simulink model "blockset_Q36121333"  (R2023a)
settings: Solver=VariableStepAuto  StartTime=0.0  StopTime=0.002  FixedStep=2e-12  MaxStep=1e-7  RelTol=1e-3
undefined symbols (not defined in the file or in its folder): plecs
libraries: plecslib_extras2 x5, simulink x5
settings Model: Creator=stanl  LastModifiedBy=stanl
settings SolverCC: ConsecutiveZCsStepRelTol=10*1280*eps
settings DataIOCC: ReturnWorkspaceOutputs=off

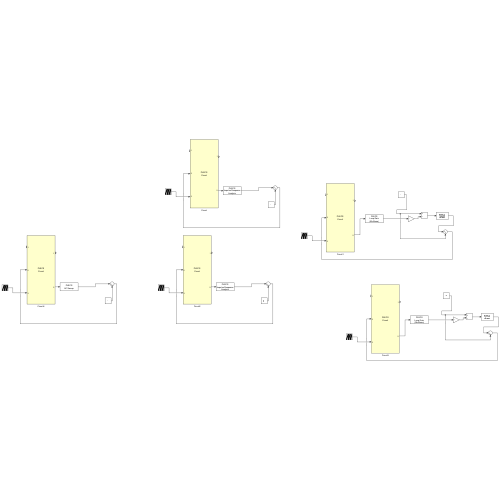
[thumbnail: Simulink's stored preview of the top-level diagram]
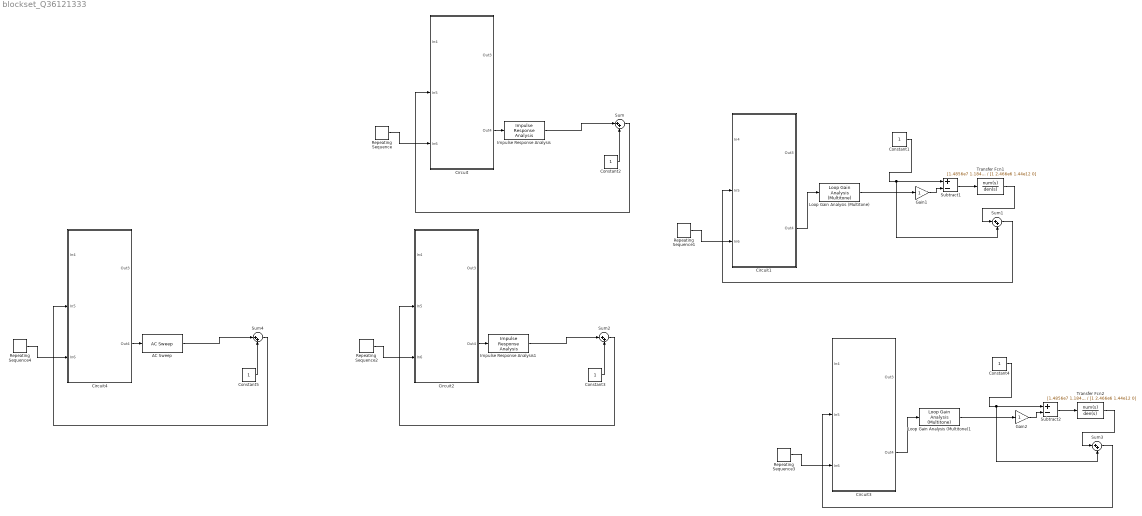
== system blockset_Q36121333 ==
  AC Sweep : plecslib_extras2/Analysis Tools/AC Sweep  FreqRange=[100 500000]  FreqScale=logarithmic  NPoints=21  InitialAmplitude=1e-3  TimeSpan=2e-6  TStart=0  ShowRefInput=off  Method=Steady-state analysis - start from model initial state  MaxIter=20  Tolerance=1e-4  Display=final  HideScopes=off  HiddenStates=error  OutputName=T  BodePlot=on  JPert=1e-4  NInitCycles=0
      settings: SourceProductName=PLECS Extras
  Circuit : Subsystem  LoadFcn=plecs('sl', 200);  InitFcn=plecs('sl', 214);  StartFcn=plecs('sl', 208);  StopFcn=plecs('sl', 209);  mask(PlecsCircuit){PLECSData=<binary blob, 3108 chars, not shown>}
      mask prompts: PLECSData "PLECS Data (Do not delete or modify!)"
      mask init:
      | % PLACE CUSTOM INITIALIZATIONS ABOVE
      | % DO NOT REMOVE
      | plecs('sl', 215);
      | % DO NOT REMOVE
      settings: CopyFcn=plecs('sl', 203);  DeleteFcn=plecs('sl', 205);  UndoDeleteFcn=plecs('sl', 206);  PreSaveFcn=plecs('sl', 211);  PostSaveFcn=plecs('sl', 201);  NameChangeFcn=plecs('sl', 210);  DestroyFcn=plecs('sl', 207);  PreCopyFcn=plecs('sl', 216);  OpenFcn=plecs('sl', 202);  ErrorFcn=plerrorfcn
      mask Help: web(['file:///' fullfile(plecsdoc, 'creatingacircuit.html')])
      mask Display: disp('PLECS\nCircuit')
  Circuit1 : Subsystem  LoadFcn=plecs('sl', 200);  InitFcn=plecs('sl', 214);  StartFcn=plecs('sl', 208);  StopFcn=plecs('sl', 209);  mask(PlecsCircuit){PLECSData=<binary blob, 3100 chars, not shown>}
      mask prompts: PLECSData "PLECS Data (Do not delete or modify!)"
      mask init:
      | % PLACE CUSTOM INITIALIZATIONS ABOVE
      | % DO NOT REMOVE
      | plecs('sl', 215);
      | % DO NOT REMOVE
      settings: CopyFcn=plecs('sl', 203);  DeleteFcn=plecs('sl', 205);  UndoDeleteFcn=plecs('sl', 206);  PreSaveFcn=plecs('sl', 211);  PostSaveFcn=plecs('sl', 201);  NameChangeFcn=plecs('sl', 210);  DestroyFcn=plecs('sl', 207);  PreCopyFcn=plecs('sl', 216);  OpenFcn=plecs('sl', 202);  ErrorFcn=plerrorfcn
      mask Help: web(['file:///' fullfile(plecsdoc, 'creatingacircuit.html')])
      mask Display: disp('PLECS\nCircuit')
  Circuit2 : Subsystem  LoadFcn=plecs('sl', 200);  InitFcn=plecs('sl', 214);  StartFcn=plecs('sl', 208);  StopFcn=plecs('sl', 209);  mask(PlecsCircuit){PLECSData=<binary blob, 3112 chars, not shown>}
      mask prompts: PLECSData "PLECS Data (Do not delete or modify!)"
      mask init:
      | % PLACE CUSTOM INITIALIZATIONS ABOVE
      | % DO NOT REMOVE
      | plecs('sl', 215);
      | % DO NOT REMOVE
      settings: CopyFcn=plecs('sl', 203);  DeleteFcn=plecs('sl', 205);  UndoDeleteFcn=plecs('sl', 206);  PreSaveFcn=plecs('sl', 211);  PostSaveFcn=plecs('sl', 201);  NameChangeFcn=plecs('sl', 210);  DestroyFcn=plecs('sl', 207);  PreCopyFcn=plecs('sl', 216);  OpenFcn=plecs('sl', 202);  ErrorFcn=plerrorfcn
      mask Help: web(['file:///' fullfile(plecsdoc, 'creatingacircuit.html')])
      mask Display: disp('PLECS\nCircuit')
  Circuit3 : Subsystem  LoadFcn=plecs('sl', 200);  InitFcn=plecs('sl', 214);  StartFcn=plecs('sl', 208);  StopFcn=plecs('sl', 209);  mask(PlecsCircuit){PLECSData=<binary blob, 3096 chars, not shown>}
      mask prompts: PLECSData "PLECS Data (Do not delete or modify!)"
      mask init:
      | % PLACE CUSTOM INITIALIZATIONS ABOVE
      | % DO NOT REMOVE
      | plecs('sl', 215);
      | % DO NOT REMOVE
      settings: CopyFcn=plecs('sl', 203);  DeleteFcn=plecs('sl', 205);  UndoDeleteFcn=plecs('sl', 206);  PreSaveFcn=plecs('sl', 211);  PostSaveFcn=plecs('sl', 201);  NameChangeFcn=plecs('sl', 210);  DestroyFcn=plecs('sl', 207);  PreCopyFcn=plecs('sl', 216);  OpenFcn=plecs('sl', 202);  ErrorFcn=plerrorfcn
      mask Help: web(['file:///' fullfile(plecsdoc, 'creatingacircuit.html')])
      mask Display: disp('PLECS\nCircuit')
  Circuit4 : Subsystem  LoadFcn=plecs('sl', 200);  InitFcn=plecs('sl', 214);  StartFcn=plecs('sl', 208);  StopFcn=plecs('sl', 209);  mask(PlecsCircuit){PLECSData=<binary blob, 3104 chars, not shown>}
      mask prompts: PLECSData "PLECS Data (Do not delete or modify!)"
      mask init:
      | % PLACE CUSTOM INITIALIZATIONS ABOVE
      | % DO NOT REMOVE
      | plecs('sl', 215);
      | % DO NOT REMOVE
      settings: CopyFcn=plecs('sl', 203);  DeleteFcn=plecs('sl', 205);  UndoDeleteFcn=plecs('sl', 206);  PreSaveFcn=plecs('sl', 211);  PostSaveFcn=plecs('sl', 201);  NameChangeFcn=plecs('sl', 210);  DestroyFcn=plecs('sl', 207);  PreCopyFcn=plecs('sl', 216);  OpenFcn=plecs('sl', 202);  ErrorFcn=plerrorfcn
      mask Help: web(['file:///' fullfile(plecsdoc, 'creatingacircuit.html')])
      mask Display: disp('PLECS\nCircuit')
  Constant{1..5} (5 alike) : Constant
  Gain1 : Gain
  Gain2 : Gain
  Impulse Response Analysis : plecslib_extras2/Analysis Tools/Impulse Response Analysis  FreqRange=[100 200000]  FreqScale=logarithmic  NPoints=300  Perturbation=1e-3  Compensation=discrete pulse  TimeSpan=2e-6  TStart=0  MaxIter=20  Tolerance=1e-6  Display=iteration  HideScopes=on  HiddenStates=error  OutputName=T  BodePlot=on  JPert=1e-4  NInitCycles=0
      settings: SourceProductName=PLECS Extras
  Impulse Response Analysis1 : plecslib_extras2/Analysis Tools/Impulse Response Analysis  FreqRange=[100 200000]  FreqScale=logarithmic  NPoints=300  Perturbation=1e-3  Compensation=discrete pulse  TimeSpan=2e-6  TStart=0  MaxIter=20  Tolerance=1e-6  Display=iteration  HideScopes=on  HiddenStates=error  OutputName=T  BodePlot=on  JPert=1e-4  NInitCycles=0
      settings: SourceProductName=PLECS Extras
  Loop Gain Analysis (Multitone) : plecslib_extras2/Analysis Tools/Loop Gain Analysis (Multitone)  FreqRange=[100 200000]  Amplitude=1e-3  TStart=0.02  Display=final  HideScopes=off  OutputName=T  BodePlot=on
      settings: SourceProductName=PLECS Extras
  Loop Gain Analysis (Multitone)1 : plecslib_extras2/Analysis Tools/Loop Gain Analysis (Multitone)  FreqRange=[100 200000]  Amplitude=1e-3  TStart=0.02  Display=final  HideScopes=off  OutputName=T  BodePlot=on
      settings: SourceProductName=PLECS Extras
  Repeating Sequence{,1..4} (5 alike) : simulink/Sources/Repeating Sequence  rep_seq_t=[0 2e-6]  rep_seq_y=[0 3]
  Subtract1 : Sum  Inputs=+-
  Subtract2 : Sum  Inputs=+-
  Sum{,1..4} (5 alike) : Sum  Inputs=|++
  Transfer Fcn1 : TransferFcn  Numerator=[1.4856e7 1.184e12 2.289e16]  Denominator=[1 2.466e6 1.44e12 0]
  Transfer Fcn2 : TransferFcn  Numerator=[1.4856e7 1.184e12 2.289e16]  Denominator=[1 2.466e6 1.44e12 0]
  wires:
  Repeating Sequence/1 -> Circuit/3(In6)
  Sum/1 -> Circuit/2(In5)
  Gain1/1 -> Subtract1/2
  Constant1/1 -> Sum1/2, Subtract1/1
  Sum1/1 -> Circuit1/2(In5)
  Transfer Fcn1/1 -> Sum1/1
  Repeating Sequence1/1 -> Circuit1/3(In6)
  Subtract1/1 -> Transfer Fcn1/1
  Circuit/2(Out4) -> Impulse Response Analysis/1
  Constant2/1 -> Sum/2
  Impulse Response Analysis/1 -> Sum/1
  Impulse Response Analysis1/1 -> Sum2/1
  Circuit2/2(Out4) -> Impulse Response Analysis1/1
  Constant3/1 -> Sum2/2
  Repeating Sequence2/1 -> Circuit2/3(In6)
  Sum2/1 -> Circuit2/2(In5)
  Loop Gain Analysis (Multitone)/1 -> Gain1/1
  Circuit1/2(Out4) -> Loop Gain Analysis (Multitone)/1
  Constant4/1 -> Sum3/2, Subtract2/1
  Subtract2/1 -> Transfer Fcn2/1
  Repeating Sequence3/1 -> Circuit3/3(In6)
  Transfer Fcn2/1 -> Sum3/1
  Gain2/1 -> Subtract2/2
  Sum3/1 -> Circuit3/2(In5)
  Circuit3/2(Out4) -> Loop Gain Analysis (Multitone)1/1
  Loop Gain Analysis (Multitone)1/1 -> Gain2/1
  Circuit4/2(Out4) -> AC Sweep/1
  Sum4/1 -> Circuit4/2(In5)
  Repeating Sequence4/1 -> Circuit4/3(In6)
  Constant5/1 -> Sum4/2
  AC Sweep/1 -> Sum4/1

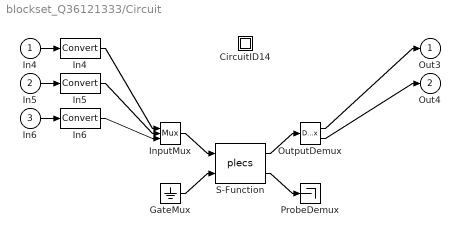
== system blockset_Q36121333/Circuit ==
  In4 : Inport  PortDimensions=1
  In5 : Inport  Port=2  PortDimensions=1
  In6 : Inport  Port=3  PortDimensions=1
  " CircuitID14 " : Subsystem
  " GateMux " : Ground
  " In4 " : DataTypeConversion
  " In5 " : DataTypeConversion
  " In6 " : DataTypeConversion
  " InputMux " : Mux  Inputs=[ 1 1 1 ]
  " OutputDemux " : Demux  Outputs=[ 1 1 ]
  " ProbeDemux " : Terminator
  " S-Function " : S-Function  FunctionName=plecs  SFunctionDeploymentMode=off  EnableBusSupport=off
  Out3 : Outport  PortDimensions=1
  Out4 : Outport  Port=2  PortDimensions=1
  wires:
  " InputMux "/1 -> " S-Function "/1
  " GateMux "/1 -> " S-Function "/2
  " S-Function "/1 -> " OutputDemux "/1
  " S-Function "/2 -> " ProbeDemux "/1
  In4/1 -> " In4 "/1
  " In4 "/1 -> " InputMux "/1
  In5/1 -> " In5 "/1
  " In5 "/1 -> " InputMux "/2
  In6/1 -> " In6 "/1
  " In6 "/1 -> " InputMux "/3
  " OutputDemux "/1 -> Out3/1
  " OutputDemux "/2 -> Out4/1

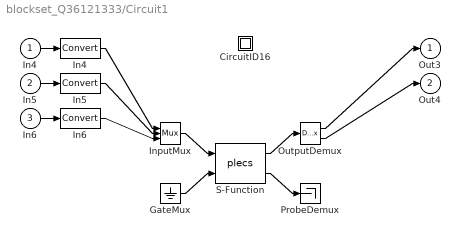
== system blockset_Q36121333/Circuit1 ==
  In4 : Inport  PortDimensions=1
  In5 : Inport  Port=2  PortDimensions=1
  In6 : Inport  Port=3  PortDimensions=1
  " CircuitID16 " : Subsystem
  " GateMux " : Ground
  " In4 " : DataTypeConversion
  " In5 " : DataTypeConversion
  " In6 " : DataTypeConversion
  " InputMux " : Mux  Inputs=[ 1 1 1 ]
  " OutputDemux " : Demux  Outputs=[ 1 1 ]
  " ProbeDemux " : Terminator
  " S-Function " : S-Function  FunctionName=plecs  SFunctionDeploymentMode=off  EnableBusSupport=off
  Out3 : Outport  PortDimensions=1
  Out4 : Outport  Port=2  PortDimensions=1
  wires:
  " InputMux "/1 -> " S-Function "/1
  " GateMux "/1 -> " S-Function "/2
  " S-Function "/1 -> " OutputDemux "/1
  " S-Function "/2 -> " ProbeDemux "/1
  In4/1 -> " In4 "/1
  " In4 "/1 -> " InputMux "/1
  In5/1 -> " In5 "/1
  " In5 "/1 -> " InputMux "/2
  In6/1 -> " In6 "/1
  " In6 "/1 -> " InputMux "/3
  " OutputDemux "/1 -> Out3/1
  " OutputDemux "/2 -> Out4/1

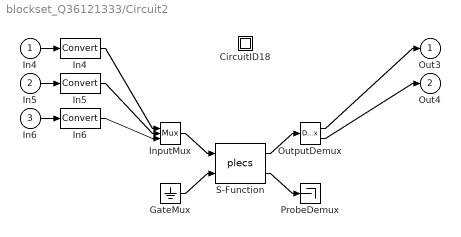
== system blockset_Q36121333/Circuit2 ==
  In4 : Inport  PortDimensions=1
  In5 : Inport  Port=2  PortDimensions=1
  In6 : Inport  Port=3  PortDimensions=1
  " CircuitID18 " : Subsystem
  " GateMux " : Ground
  " In4 " : DataTypeConversion
  " In5 " : DataTypeConversion
  " In6 " : DataTypeConversion
  " InputMux " : Mux  Inputs=[ 1 1 1 ]
  " OutputDemux " : Demux  Outputs=[ 1 1 ]
  " ProbeDemux " : Terminator
  " S-Function " : S-Function  FunctionName=plecs  SFunctionDeploymentMode=off  EnableBusSupport=off
  Out3 : Outport  PortDimensions=1
  Out4 : Outport  Port=2  PortDimensions=1
  wires:
  " InputMux "/1 -> " S-Function "/1
  " GateMux "/1 -> " S-Function "/2
  " S-Function "/1 -> " OutputDemux "/1
  " S-Function "/2 -> " ProbeDemux "/1
  In4/1 -> " In4 "/1
  " In4 "/1 -> " InputMux "/1
  In5/1 -> " In5 "/1
  " In5 "/1 -> " InputMux "/2
  In6/1 -> " In6 "/1
  " In6 "/1 -> " InputMux "/3
  " OutputDemux "/1 -> Out3/1
  " OutputDemux "/2 -> Out4/1

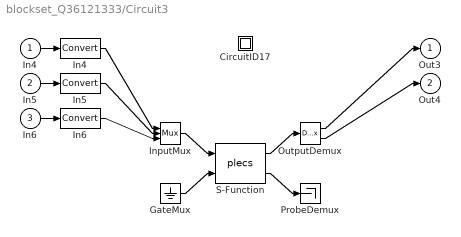
== system blockset_Q36121333/Circuit3 ==
  In4 : Inport  PortDimensions=1
  In5 : Inport  Port=2  PortDimensions=1
  In6 : Inport  Port=3  PortDimensions=1
  " CircuitID17 " : Subsystem
  " GateMux " : Ground
  " In4 " : DataTypeConversion
  " In5 " : DataTypeConversion
  " In6 " : DataTypeConversion
  " InputMux " : Mux  Inputs=[ 1 1 1 ]
  " OutputDemux " : Demux  Outputs=[ 1 1 ]
  " ProbeDemux " : Terminator
  " S-Function " : S-Function  FunctionName=plecs  SFunctionDeploymentMode=off  EnableBusSupport=off
  Out3 : Outport  PortDimensions=1
  Out4 : Outport  Port=2  PortDimensions=1
  wires:
  " InputMux "/1 -> " S-Function "/1
  " GateMux "/1 -> " S-Function "/2
  " S-Function "/1 -> " OutputDemux "/1
  " S-Function "/2 -> " ProbeDemux "/1
  In4/1 -> " In4 "/1
  " In4 "/1 -> " InputMux "/1
  In5/1 -> " In5 "/1
  " In5 "/1 -> " InputMux "/2
  In6/1 -> " In6 "/1
  " In6 "/1 -> " InputMux "/3
  " OutputDemux "/1 -> Out3/1
  " OutputDemux "/2 -> Out4/1

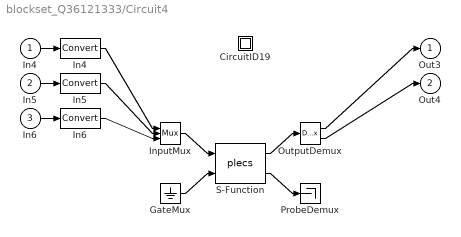
== system blockset_Q36121333/Circuit4 ==
  In4 : Inport  PortDimensions=1
  In5 : Inport  Port=2  PortDimensions=1
  In6 : Inport  Port=3  PortDimensions=1
  " CircuitID19 " : Subsystem
  " GateMux " : Ground
  " In4 " : DataTypeConversion
  " In5 " : DataTypeConversion
  " In6 " : DataTypeConversion
  " InputMux " : Mux  Inputs=[ 1 1 1 ]
  " OutputDemux " : Demux  Outputs=[ 1 1 ]
  " ProbeDemux " : Terminator
  " S-Function " : S-Function  FunctionName=plecs  SFunctionDeploymentMode=off  EnableBusSupport=off
  Out3 : Outport  PortDimensions=1
  Out4 : Outport  Port=2  PortDimensions=1
  wires:
  " InputMux "/1 -> " S-Function "/1
  " GateMux "/1 -> " S-Function "/2
  " S-Function "/1 -> " OutputDemux "/1
  " S-Function "/2 -> " ProbeDemux "/1
  In4/1 -> " In4 "/1
  " In4 "/1 -> " InputMux "/1
  In5/1 -> " In5 "/1
  " In5 "/1 -> " InputMux "/2
  In6/1 -> " In6 "/1
  " In6 "/1 -> " InputMux "/3
  " OutputDemux "/1 -> Out3/1
  " OutputDemux "/2 -> Out4/1

== system blockset_Q36121333/Circuit/ CircuitID14  ==

== system blockset_Q36121333/Circuit1/ CircuitID16  ==

== system blockset_Q36121333/Circuit2/ CircuitID18  ==

== system blockset_Q36121333/Circuit3/ CircuitID17  ==

== system blockset_Q36121333/Circuit4/ CircuitID19  ==
